simulink model "Model_with_decision"  (R2022a)
settings: Solver=VariableStepAuto  StartTime=0.0  StopTime=1000000  RelTol=1e-3
undefined symbols (not defined in the file): Coefficient_value, Enable_X, Enable_Y, N, s1, s10, s11, s12, s13, s14, s15, s16, s17, s18, s19, s2, s20, s21, s22, s23, s24, s25, s26, s27, s28, s29, s3, s30, s4, s5, s6, s7, s8, s9
libraries: simulink x35
(part 2 of 5)

== system Model_with_decision/Pbit_14 ==
  note: so EN=0 block simply passes the same OUT value to a multiport switch
  note: random value does not change when EN=0
  note: without a delay block, this block naturally gets the output of EN=1 block's output @ EN=0 so an unit delay is naturally applied
  IN : Inport
  EN : Inport  Port=2
  Cast To Double : DataTypeConversion  OutDataTypeStr=double  SaturateOnIntegerOverflow=off  RndMeth=Floor
  Cast To Double1 : DataTypeConversion  OutDataTypeStr=double  SaturateOnIntegerOverflow=off  RndMeth=Floor
  EN=0 Block : Subsystem  TreatAsAtomicUnit=on
  EN=1 Block : Subsystem  TreatAsAtomicUnit=on
  If : If
  Multiport Switch : MultiPortSwitch  DataPortOrder=Zero-based contiguous  Inputs=2  zeroidx=on  SaturateOnIntegerOverflow=off  InputSameDT=off
  OUT : Outport
  wires:
  IN/1 -> EN=1 Block/1(IN)
  EN/1 -> [EN], If/1
  Multiport Switch/1 -> OUT/1  "OUT_MUX"
  If/1 -> EN=1 Block/Action
  If/2 -> EN=0 Block/Action
  EN=1 Block/1(OUT) -> Cast To Double/1, EN=0 Block/1(IN)  "OUT_EN=1"
  EN=0 Block/1(Out1) -> Cast To Double1/1  "OUT_EN=0"
  [EN] -> Multiport Switch/1
  Cast To Double/1 -> Multiport Switch/3
  Cast To Double1/1 -> Multiport Switch/2

== system Model_with_decision/Pbit_15 ==
  note: without a delay block, this block naturally gets the output of EN=1 block's output @ EN=0 so an unit delay is naturally applied
  note: random value does not change when EN=0
  note: so EN=0 block simply passes the same OUT value to a multiport switch
  IN : Inport
  EN : Inport  Port=2
  Cast To Double : DataTypeConversion  OutDataTypeStr=double  SaturateOnIntegerOverflow=off  RndMeth=Floor
  Cast To Double1 : DataTypeConversion  OutDataTypeStr=double  SaturateOnIntegerOverflow=off  RndMeth=Floor
  EN=0 Block : Subsystem  TreatAsAtomicUnit=on
  EN=1 Block : Subsystem  TreatAsAtomicUnit=on
  If : If
  Multiport Switch : MultiPortSwitch  DataPortOrder=Zero-based contiguous  Inputs=2  zeroidx=on  SaturateOnIntegerOverflow=off  InputSameDT=off
  OUT : Outport
  wires:
  Cast To Double1/1 -> Multiport Switch/2
  Cast To Double/1 -> Multiport Switch/3
  [EN] -> Multiport Switch/1
  EN=0 Block/1(Out1) -> Cast To Double1/1  "OUT_EN=0"
  EN=1 Block/1(OUT) -> EN=0 Block/1(IN), Cast To Double/1  "OUT_EN=1"
  If/2 -> EN=0 Block/Action
  If/1 -> EN=1 Block/Action
  Multiport Switch/1 -> OUT/1  "OUT_MUX"
  EN/1 -> If/1, [EN]
  IN/1 -> EN=1 Block/1(IN)

== system Model_with_decision/Pbit_2 ==
  note: without a delay block, this block naturally gets the output of EN=1 block's output @ EN=0 so an unit delay is naturally applied
  note: random value does not change when EN=0
  note: so EN=0 block simply passes the same OUT value to a multiport switch
  IN : Inport
  EN : Inport  Port=2
  Cast To Double : DataTypeConversion  OutDataTypeStr=double  SaturateOnIntegerOverflow=off  RndMeth=Floor
  Cast To Double1 : DataTypeConversion  OutDataTypeStr=double  SaturateOnIntegerOverflow=off  RndMeth=Floor
  EN=0 Block : Subsystem  TreatAsAtomicUnit=on
  EN=1 Block : Subsystem  TreatAsAtomicUnit=on
  If : If
  Multiport Switch : MultiPortSwitch  DataPortOrder=Zero-based contiguous  Inputs=2  zeroidx=on  SaturateOnIntegerOverflow=off  InputSameDT=off
  OUT : Outport
  wires:
  Cast To Double1/1 -> Multiport Switch/2
  Cast To Double/1 -> Multiport Switch/3
  [EN] -> Multiport Switch/1
  EN=0 Block/1(Out1) -> Cast To Double1/1  "OUT_EN=0"
  EN=1 Block/1(OUT) -> EN=0 Block/1(IN), Cast To Double/1  "OUT_EN=1"
  If/2 -> EN=0 Block/Action
  If/1 -> EN=1 Block/Action
  Multiport Switch/1 -> OUT/1  "OUT_MUX"
  EN/1 -> If/1, [EN]
  IN/1 -> EN=1 Block/1(IN)

== system Model_with_decision/Pbit_3 ==
  note: so EN=0 block simply passes the same OUT value to a multiport switch
  note: random value does not change when EN=0
  note: without a delay block, this block naturally gets the output of EN=1 block's output @ EN=0 so an unit delay is naturally applied
  IN : Inport
  EN : Inport  Port=2
  Cast To Double : DataTypeConversion  OutDataTypeStr=double  SaturateOnIntegerOverflow=off  RndMeth=Floor
  Cast To Double1 : DataTypeConversion  OutDataTypeStr=double  SaturateOnIntegerOverflow=off  RndMeth=Floor
  EN=0 Block : Subsystem  TreatAsAtomicUnit=on
  EN=1 Block : Subsystem  TreatAsAtomicUnit=on
  If : If
  Multiport Switch : MultiPortSwitch  DataPortOrder=Zero-based contiguous  Inputs=2  zeroidx=on  SaturateOnIntegerOverflow=off  InputSameDT=off
  OUT : Outport
  wires:
  IN/1 -> EN=1 Block/1(IN)
  EN/1 -> [EN], If/1
  Multiport Switch/1 -> OUT/1  "OUT_MUX"
  If/1 -> EN=1 Block/Action
  If/2 -> EN=0 Block/Action
  EN=1 Block/1(OUT) -> Cast To Double/1, EN=0 Block/1(IN)  "OUT_EN=1"
  EN=0 Block/1(Out1) -> Cast To Double1/1  "OUT_EN=0"
  [EN] -> Multiport Switch/1
  Cast To Double/1 -> Multiport Switch/3
  Cast To Double1/1 -> Multiport Switch/2

== system Model_with_decision/Pbit_4 ==
  note: so EN=0 block simply passes the same OUT value to a multiport switch
  note: random value does not change when EN=0
  note: without a delay block, this block naturally gets the output of EN=1 block's output @ EN=0 so an unit delay is naturally applied
  IN : Inport
  EN : Inport  Port=2
  Cast To Double : DataTypeConversion  OutDataTypeStr=double  SaturateOnIntegerOverflow=off  RndMeth=Floor
  Cast To Double1 : DataTypeConversion  OutDataTypeStr=double  SaturateOnIntegerOverflow=off  RndMeth=Floor
  EN=0 Block : Subsystem  TreatAsAtomicUnit=on
  EN=1 Block : Subsystem  TreatAsAtomicUnit=on
  If : If
  Multiport Switch : MultiPortSwitch  DataPortOrder=Zero-based contiguous  Inputs=2  zeroidx=on  SaturateOnIntegerOverflow=off  InputSameDT=off
  OUT : Outport
  wires:
  IN/1 -> EN=1 Block/1(IN)
  EN/1 -> [EN], If/1
  Multiport Switch/1 -> OUT/1  "OUT_MUX"
  If/1 -> EN=1 Block/Action
  If/2 -> EN=0 Block/Action
  EN=1 Block/1(OUT) -> Cast To Double/1, EN=0 Block/1(IN)  "OUT_EN=1"
  EN=0 Block/1(Out1) -> Cast To Double1/1  "OUT_EN=0"
  [EN] -> Multiport Switch/1
  Cast To Double/1 -> Multiport Switch/3
  Cast To Double1/1 -> Multiport Switch/2

== system Model_with_decision/Pbit_5 ==
  note: without a delay block, this block naturally gets the output of EN=1 block's output @ EN=0 so an unit delay is naturally applied
  note: random value does not change when EN=0
  note: so EN=0 block simply passes the same OUT value to a multiport switch
  IN : Inport
  EN : Inport  Port=2
  Cast To Double : DataTypeConversion  OutDataTypeStr=double  SaturateOnIntegerOverflow=off  RndMeth=Floor
  Cast To Double1 : DataTypeConversion  OutDataTypeStr=double  SaturateOnIntegerOverflow=off  RndMeth=Floor
  EN=0 Block : Subsystem  TreatAsAtomicUnit=on
  EN=1 Block : Subsystem  TreatAsAtomicUnit=on
  If : If
  Multiport Switch : MultiPortSwitch  DataPortOrder=Zero-based contiguous  Inputs=2  zeroidx=on  SaturateOnIntegerOverflow=off  InputSameDT=off
  OUT : Outport
  wires:
  Cast To Double1/1 -> Multiport Switch/2
  Cast To Double/1 -> Multiport Switch/3
  [EN] -> Multiport Switch/1
  EN=0 Block/1(Out1) -> Cast To Double1/1  "OUT_EN=0"
  EN=1 Block/1(OUT) -> EN=0 Block/1(IN), Cast To Double/1  "OUT_EN=1"
  If/2 -> EN=0 Block/Action
  If/1 -> EN=1 Block/Action
  Multiport Switch/1 -> OUT/1  "OUT_MUX"
  EN/1 -> If/1, [EN]
  IN/1 -> EN=1 Block/1(IN)

== system Model_with_decision/Pbit_6 ==
  note: without a delay block, this block naturally gets the output of EN=1 block's output @ EN=0 so an unit delay is naturally applied
  note: random value does not change when EN=0
  note: so EN=0 block simply passes the same OUT value to a multiport switch
  IN : Inport
  EN : Inport  Port=2
  Cast To Double : DataTypeConversion  OutDataTypeStr=double  SaturateOnIntegerOverflow=off  RndMeth=Floor
  Cast To Double1 : DataTypeConversion  OutDataTypeStr=double  SaturateOnIntegerOverflow=off  RndMeth=Floor
  EN=0 Block : Subsystem  TreatAsAtomicUnit=on
  EN=1 Block : Subsystem  TreatAsAtomicUnit=on
  If : If
  Multiport Switch : MultiPortSwitch  DataPortOrder=Zero-based contiguous  Inputs=2  zeroidx=on  SaturateOnIntegerOverflow=off  InputSameDT=off
  OUT : Outport
  wires:
  Cast To Double1/1 -> Multiport Switch/2
  Cast To Double/1 -> Multiport Switch/3
  [EN] -> Multiport Switch/1
  EN=0 Block/1(Out1) -> Cast To Double1/1  "OUT_EN=0"
  EN=1 Block/1(OUT) -> EN=0 Block/1(IN), Cast To Double/1  "OUT_EN=1"
  If/2 -> EN=0 Block/Action
  If/1 -> EN=1 Block/Action
  Multiport Switch/1 -> OUT/1  "OUT_MUX"
  EN/1 -> If/1, [EN]
  IN/1 -> EN=1 Block/1(IN)

== system Model_with_decision/Pbit_7 ==
  note: without a delay block, this block naturally gets the output of EN=1 block's output @ EN=0 so an unit delay is naturally applied
  note: random value does not change when EN=0
  note: so EN=0 block simply passes the same OUT value to a multiport switch
  IN : Inport
  EN : Inport  Port=2
  Cast To Double : DataTypeConversion  OutDataTypeStr=double  SaturateOnIntegerOverflow=off  RndMeth=Floor
  Cast To Double1 : DataTypeConversion  OutDataTypeStr=double  SaturateOnIntegerOverflow=off  RndMeth=Floor
  EN=0 Block : Subsystem  TreatAsAtomicUnit=on
  EN=1 Block : Subsystem  TreatAsAtomicUnit=on
  If : If
  Multiport Switch : MultiPortSwitch  DataPortOrder=Zero-based contiguous  Inputs=2  zeroidx=on  SaturateOnIntegerOverflow=off  InputSameDT=off
  OUT : Outport
  wires:
  Cast To Double1/1 -> Multiport Switch/2
  Cast To Double/1 -> Multiport Switch/3
  [EN] -> Multiport Switch/1
  EN=0 Block/1(Out1) -> Cast To Double1/1  "OUT_EN=0"
  EN=1 Block/1(OUT) -> EN=0 Block/1(IN), Cast To Double/1  "OUT_EN=1"
  If/2 -> EN=0 Block/Action
  If/1 -> EN=1 Block/Action
  Multiport Switch/1 -> OUT/1  "OUT_MUX"
  EN/1 -> If/1, [EN]
  IN/1 -> EN=1 Block/1(IN)

== system Model_with_decision/Pbit_8 ==
  note: so EN=0 block simply passes the same OUT value to a multiport switch
  note: random value does not change when EN=0
  note: without a delay block, this block naturally gets the output of EN=1 block's output @ EN=0 so an unit delay is naturally applied
  IN : Inport
  EN : Inport  Port=2
  Cast To Double : DataTypeConversion  OutDataTypeStr=double  SaturateOnIntegerOverflow=off  RndMeth=Floor
  Cast To Double1 : DataTypeConversion  OutDataTypeStr=double  SaturateOnIntegerOverflow=off  RndMeth=Floor
  EN=0 Block : Subsystem  TreatAsAtomicUnit=on
  EN=1 Block : Subsystem  TreatAsAtomicUnit=on
  If : If
  Multiport Switch : MultiPortSwitch  DataPortOrder=Zero-based contiguous  Inputs=2  zeroidx=on  SaturateOnIntegerOverflow=off  InputSameDT=off
  OUT : Outport
  wires:
  IN/1 -> EN=1 Block/1(IN)
  EN/1 -> [EN], If/1
  Multiport Switch/1 -> OUT/1  "OUT_MUX"
  If/1 -> EN=1 Block/Action
  If/2 -> EN=0 Block/Action
  EN=1 Block/1(OUT) -> Cast To Double/1, EN=0 Block/1(IN)  "OUT_EN=1"
  EN=0 Block/1(Out1) -> Cast To Double1/1  "OUT_EN=0"
  [EN] -> Multiport Switch/1
  Cast To Double/1 -> Multiport Switch/3
  Cast To Double1/1 -> Multiport Switch/2

== system Model_with_decision/Pbit_9 ==
  note: so EN=0 block simply passes the same OUT value to a multiport switch
  note: random value does not change when EN=0
  note: without a delay block, this block naturally gets the output of EN=1 block's output @ EN=0 so an unit delay is naturally applied
  IN : Inport
  EN : Inport  Port=2
  Cast To Double : DataTypeConversion  OutDataTypeStr=double  SaturateOnIntegerOverflow=off  RndMeth=Floor
  Cast To Double1 : DataTypeConversion  OutDataTypeStr=double  SaturateOnIntegerOverflow=off  RndMeth=Floor
  EN=0 Block : Subsystem  TreatAsAtomicUnit=on
  EN=1 Block : Subsystem  TreatAsAtomicUnit=on
  If : If
  Multiport Switch : MultiPortSwitch  DataPortOrder=Zero-based contiguous  Inputs=2  zeroidx=on  SaturateOnIntegerOverflow=off  InputSameDT=off
  OUT : Outport
  wires:
  IN/1 -> EN=1 Block/1(IN)
  EN/1 -> [EN], If/1
  Multiport Switch/1 -> OUT/1  "OUT_MUX"
  If/1 -> EN=1 Block/Action
  If/2 -> EN=0 Block/Action
  EN=1 Block/1(OUT) -> Cast To Double/1, EN=0 Block/1(IN)  "OUT_EN=1"
  EN=0 Block/1(Out1) -> Cast To Double1/1  "OUT_EN=0"
  [EN] -> Multiport Switch/1
  Cast To Double/1 -> Multiport Switch/3
  Cast To Double1/1 -> Multiport Switch/2

== system Model_with_decision/Pbit_Y_1 ==
  note: without a delay block, this block naturally gets the output of EN=1 block's output @ EN=0 so an unit delay is naturally applied
  note: random value does not change when EN=0
  note: so EN=0 block simply passes the same OUT value to a multiport switch
  IN : Inport
  EN : Inport  Port=2
  Cast To Double : DataTypeConversion  OutDataTypeStr=double  SaturateOnIntegerOverflow=off  RndMeth=Floor
  Cast To Double1 : DataTypeConversion  OutDataTypeStr=double  SaturateOnIntegerOverflow=off  RndMeth=Floor
  EN=0 Block : Subsystem  TreatAsAtomicUnit=on
  EN=1 Block : Subsystem  TreatAsAtomicUnit=on
  If : If
  Multiport Switch : MultiPortSwitch  DataPortOrder=Zero-based contiguous  Inputs=2  zeroidx=on  SaturateOnIntegerOverflow=off  InputSameDT=off
  OUT : Outport
  wires:
  Cast To Double1/1 -> Multiport Switch/2
  Cast To Double/1 -> Multiport Switch/3
  [EN] -> Multiport Switch/1
  EN=0 Block/1(Out1) -> Cast To Double1/1  "OUT_EN=0"
  EN=1 Block/1(OUT) -> EN=0 Block/1(IN), Cast To Double/1  "OUT_EN=1"
  If/2 -> EN=0 Block/Action
  If/1 -> EN=1 Block/Action
  Multiport Switch/1 -> OUT/1  "OUT_MUX"
  EN/1 -> If/1, [EN]
  IN/1 -> EN=1 Block/1(IN)

== system Model_with_decision/Pbit_Y_10 ==
  note: without a delay block, this block naturally gets the output of EN=1 block's output @ EN=0 so an unit delay is naturally applied
  note: random value does not change when EN=0
  note: so EN=0 block simply passes the same OUT value to a multiport switch
  IN : Inport
  EN : Inport  Port=2
  Cast To Double : DataTypeConversion  OutDataTypeStr=double  SaturateOnIntegerOverflow=off  RndMeth=Floor
  Cast To Double1 : DataTypeConversion  OutDataTypeStr=double  SaturateOnIntegerOverflow=off  RndMeth=Floor
  EN=0 Block : Subsystem  TreatAsAtomicUnit=on
  EN=1 Block : Subsystem  TreatAsAtomicUnit=on
  If : If
  Multiport Switch : MultiPortSwitch  DataPortOrder=Zero-based contiguous  Inputs=2  zeroidx=on  SaturateOnIntegerOverflow=off  InputSameDT=off
  OUT : Outport
  wires:
  Cast To Double1/1 -> Multiport Switch/2
  Cast To Double/1 -> Multiport Switch/3
  [EN] -> Multiport Switch/1
  EN=0 Block/1(Out1) -> Cast To Double1/1  "OUT_EN=0"
  EN=1 Block/1(OUT) -> EN=0 Block/1(IN), Cast To Double/1  "OUT_EN=1"
  If/2 -> EN=0 Block/Action
  If/1 -> EN=1 Block/Action
  Multiport Switch/1 -> OUT/1  "OUT_MUX"
  EN/1 -> If/1, [EN]
  IN/1 -> EN=1 Block/1(IN)

== system Model_with_decision/Pbit_Y_11 ==
  note: without a delay block, this block naturally gets the output of EN=1 block's output @ EN=0 so an unit delay is naturally applied
  note: random value does not change when EN=0
  note: so EN=0 block simply passes the same OUT value to a multiport switch
  IN : Inport
  EN : Inport  Port=2
  Cast To Double : DataTypeConversion  OutDataTypeStr=double  SaturateOnIntegerOverflow=off  RndMeth=Floor
  Cast To Double1 : DataTypeConversion  OutDataTypeStr=double  SaturateOnIntegerOverflow=off  RndMeth=Floor
  EN=0 Block : Subsystem  TreatAsAtomicUnit=on
  EN=1 Block : Subsystem  TreatAsAtomicUnit=on
  If : If
  Multiport Switch : MultiPortSwitch  DataPortOrder=Zero-based contiguous  Inputs=2  zeroidx=on  SaturateOnIntegerOverflow=off  InputSameDT=off
  OUT : Outport
  wires:
  Cast To Double1/1 -> Multiport Switch/2
  Cast To Double/1 -> Multiport Switch/3
  [EN] -> Multiport Switch/1
  EN=0 Block/1(Out1) -> Cast To Double1/1  "OUT_EN=0"
  EN=1 Block/1(OUT) -> EN=0 Block/1(IN), Cast To Double/1  "OUT_EN=1"
  If/2 -> EN=0 Block/Action
  If/1 -> EN=1 Block/Action
  Multiport Switch/1 -> OUT/1  "OUT_MUX"
  EN/1 -> If/1, [EN]
  IN/1 -> EN=1 Block/1(IN)

== system Model_with_decision/Pbit_Y_12 ==
  note: without a delay block, this block naturally gets the output of EN=1 block's output @ EN=0 so an unit delay is naturally applied
  note: random value does not change when EN=0
  note: so EN=0 block simply passes the same OUT value to a multiport switch
  IN : Inport
  EN : Inport  Port=2
  Cast To Double : DataTypeConversion  OutDataTypeStr=double  SaturateOnIntegerOverflow=off  RndMeth=Floor
  Cast To Double1 : DataTypeConversion  OutDataTypeStr=double  SaturateOnIntegerOverflow=off  RndMeth=Floor
  EN=0 Block : Subsystem  TreatAsAtomicUnit=on
  EN=1 Block : Subsystem  TreatAsAtomicUnit=on
  If : If
  Multiport Switch : MultiPortSwitch  DataPortOrder=Zero-based contiguous  Inputs=2  zeroidx=on  SaturateOnIntegerOverflow=off  InputSameDT=off
  OUT : Outport
  wires:
  Cast To Double1/1 -> Multiport Switch/2
  Cast To Double/1 -> Multiport Switch/3
  [EN] -> Multiport Switch/1
  EN=0 Block/1(Out1) -> Cast To Double1/1  "OUT_EN=0"
  EN=1 Block/1(OUT) -> EN=0 Block/1(IN), Cast To Double/1  "OUT_EN=1"
  If/2 -> EN=0 Block/Action
  If/1 -> EN=1 Block/Action
  Multiport Switch/1 -> OUT/1  "OUT_MUX"
  EN/1 -> If/1, [EN]
  IN/1 -> EN=1 Block/1(IN)

== system Model_with_decision/Pbit_Y_13 ==
  note: so EN=0 block simply passes the same OUT value to a multiport switch
  note: random value does not change when EN=0
  note: without a delay block, this block naturally gets the output of EN=1 block's output @ EN=0 so an unit delay is naturally applied
  IN : Inport
  EN : Inport  Port=2
  Cast To Double : DataTypeConversion  OutDataTypeStr=double  SaturateOnIntegerOverflow=off  RndMeth=Floor
  Cast To Double1 : DataTypeConversion  OutDataTypeStr=double  SaturateOnIntegerOverflow=off  RndMeth=Floor
  EN=0 Block : Subsystem  TreatAsAtomicUnit=on
  EN=1 Block : Subsystem  TreatAsAtomicUnit=on
  If : If
  Multiport Switch : MultiPortSwitch  DataPortOrder=Zero-based contiguous  Inputs=2  zeroidx=on  SaturateOnIntegerOverflow=off  InputSameDT=off
  OUT : Outport
  wires:
  IN/1 -> EN=1 Block/1(IN)
  EN/1 -> [EN], If/1
  Multiport Switch/1 -> OUT/1  "OUT_MUX"
  If/1 -> EN=1 Block/Action
  If/2 -> EN=0 Block/Action
  EN=1 Block/1(OUT) -> Cast To Double/1, EN=0 Block/1(IN)  "OUT_EN=1"
  EN=0 Block/1(Out1) -> Cast To Double1/1  "OUT_EN=0"
  [EN] -> Multiport Switch/1
  Cast To Double/1 -> Multiport Switch/3
  Cast To Double1/1 -> Multiport Switch/2

== system Model_with_decision/Pbit_Y_14 ==
  note: so EN=0 block simply passes the same OUT value to a multiport switch
  note: random value does not change when EN=0
  note: without a delay block, this block naturally gets the output of EN=1 block's output @ EN=0 so an unit delay is naturally applied
  IN : Inport
  EN : Inport  Port=2
  Cast To Double : DataTypeConversion  OutDataTypeStr=double  SaturateOnIntegerOverflow=off  RndMeth=Floor
  Cast To Double1 : DataTypeConversion  OutDataTypeStr=double  SaturateOnIntegerOverflow=off  RndMeth=Floor
  EN=0 Block : Subsystem  TreatAsAtomicUnit=on
  EN=1 Block : Subsystem  TreatAsAtomicUnit=on
  If : If
  Multiport Switch : MultiPortSwitch  DataPortOrder=Zero-based contiguous  Inputs=2  zeroidx=on  SaturateOnIntegerOverflow=off  InputSameDT=off
  OUT : Outport
  wires:
  IN/1 -> EN=1 Block/1(IN)
  EN/1 -> [EN], If/1
  Multiport Switch/1 -> OUT/1  "OUT_MUX"
  If/1 -> EN=1 Block/Action
  If/2 -> EN=0 Block/Action
  EN=1 Block/1(OUT) -> Cast To Double/1, EN=0 Block/1(IN)  "OUT_EN=1"
  EN=0 Block/1(Out1) -> Cast To Double1/1  "OUT_EN=0"
  [EN] -> Multiport Switch/1
  Cast To Double/1 -> Multiport Switch/3
  Cast To Double1/1 -> Multiport Switch/2

== system Model_with_decision/Pbit_Y_15 ==
  note: so EN=0 block simply passes the same OUT value to a multiport switch
  note: random value does not change when EN=0
  note: without a delay block, this block naturally gets the output of EN=1 block's output @ EN=0 so an unit delay is naturally applied
  IN : Inport
  EN : Inport  Port=2
  Cast To Double : DataTypeConversion  OutDataTypeStr=double  SaturateOnIntegerOverflow=off  RndMeth=Floor
  Cast To Double1 : DataTypeConversion  OutDataTypeStr=double  SaturateOnIntegerOverflow=off  RndMeth=Floor
  EN=0 Block : Subsystem  TreatAsAtomicUnit=on
  EN=1 Block : Subsystem  TreatAsAtomicUnit=on
  If : If
  Multiport Switch : MultiPortSwitch  DataPortOrder=Zero-based contiguous  Inputs=2  zeroidx=on  SaturateOnIntegerOverflow=off  InputSameDT=off
  OUT : Outport
  wires:
  IN/1 -> EN=1 Block/1(IN)
  EN/1 -> [EN], If/1
  Multiport Switch/1 -> OUT/1  "OUT_MUX"
  If/1 -> EN=1 Block/Action
  If/2 -> EN=0 Block/Action
  EN=1 Block/1(OUT) -> Cast To Double/1, EN=0 Block/1(IN)  "OUT_EN=1"
  EN=0 Block/1(Out1) -> Cast To Double1/1  "OUT_EN=0"
  [EN] -> Multiport Switch/1
  Cast To Double/1 -> Multiport Switch/3
  Cast To Double1/1 -> Multiport Switch/2

== system Model_with_decision/Pbit_Y_2 ==
  note: without a delay block, this block naturally gets the output of EN=1 block's output @ EN=0 so an unit delay is naturally applied
  note: random value does not change when EN=0
  note: so EN=0 block simply passes the same OUT value to a multiport switch
  IN : Inport
  EN : Inport  Port=2
  Cast To Double : DataTypeConversion  OutDataTypeStr=double  SaturateOnIntegerOverflow=off  RndMeth=Floor
  Cast To Double1 : DataTypeConversion  OutDataTypeStr=double  SaturateOnIntegerOverflow=off  RndMeth=Floor
  EN=0 Block : Subsystem  TreatAsAtomicUnit=on
  EN=1 Block : Subsystem  TreatAsAtomicUnit=on
  If : If
  Multiport Switch : MultiPortSwitch  DataPortOrder=Zero-based contiguous  Inputs=2  zeroidx=on  SaturateOnIntegerOverflow=off  InputSameDT=off
  OUT : Outport
  wires:
  Cast To Double1/1 -> Multiport Switch/2
  Cast To Double/1 -> Multiport Switch/3
  [EN] -> Multiport Switch/1
  EN=0 Block/1(Out1) -> Cast To Double1/1  "OUT_EN=0"
  EN=1 Block/1(OUT) -> EN=0 Block/1(IN), Cast To Double/1  "OUT_EN=1"
  If/2 -> EN=0 Block/Action
  If/1 -> EN=1 Block/Action
  Multiport Switch/1 -> OUT/1  "OUT_MUX"
  EN/1 -> If/1, [EN]
  IN/1 -> EN=1 Block/1(IN)

== system Model_with_decision/Pbit_Y_3 ==
  note: so EN=0 block simply passes the same OUT value to a multiport switch
  note: random value does not change when EN=0
  note: without a delay block, this block naturally gets the output of EN=1 block's output @ EN=0 so an unit delay is naturally applied
  IN : Inport
  EN : Inport  Port=2
  Cast To Double : DataTypeConversion  OutDataTypeStr=double  SaturateOnIntegerOverflow=off  RndMeth=Floor
  Cast To Double1 : DataTypeConversion  OutDataTypeStr=double  SaturateOnIntegerOverflow=off  RndMeth=Floor
  EN=0 Block : Subsystem  TreatAsAtomicUnit=on
  EN=1 Block : Subsystem  TreatAsAtomicUnit=on
  If : If
  Multiport Switch : MultiPortSwitch  DataPortOrder=Zero-based contiguous  Inputs=2  zeroidx=on  SaturateOnIntegerOverflow=off  InputSameDT=off
  OUT : Outport
  wires:
  IN/1 -> EN=1 Block/1(IN)
  EN/1 -> [EN], If/1
  Multiport Switch/1 -> OUT/1  "OUT_MUX"
  If/1 -> EN=1 Block/Action
  If/2 -> EN=0 Block/Action
  EN=1 Block/1(OUT) -> Cast To Double/1, EN=0 Block/1(IN)  "OUT_EN=1"
  EN=0 Block/1(Out1) -> Cast To Double1/1  "OUT_EN=0"
  [EN] -> Multiport Switch/1
  Cast To Double/1 -> Multiport Switch/3
  Cast To Double1/1 -> Multiport Switch/2

== system Model_with_decision/Pbit_Y_4 ==
  note: so EN=0 block simply passes the same OUT value to a multiport switch
  note: random value does not change when EN=0
  note: without a delay block, this block naturally gets the output of EN=1 block's output @ EN=0 so an unit delay is naturally applied
  IN : Inport
  EN : Inport  Port=2
  Cast To Double : DataTypeConversion  OutDataTypeStr=double  SaturateOnIntegerOverflow=off  RndMeth=Floor
  Cast To Double1 : DataTypeConversion  OutDataTypeStr=double  SaturateOnIntegerOverflow=off  RndMeth=Floor
  EN=0 Block : Subsystem  TreatAsAtomicUnit=on
  EN=1 Block : Subsystem  TreatAsAtomicUnit=on
  If : If
  Multiport Switch : MultiPortSwitch  DataPortOrder=Zero-based contiguous  Inputs=2  zeroidx=on  SaturateOnIntegerOverflow=off  InputSameDT=off
  OUT : Outport
  wires:
  IN/1 -> EN=1 Block/1(IN)
  EN/1 -> [EN], If/1
  Multiport Switch/1 -> OUT/1  "OUT_MUX"
  If/1 -> EN=1 Block/Action
  If/2 -> EN=0 Block/Action
  EN=1 Block/1(OUT) -> Cast To Double/1, EN=0 Block/1(IN)  "OUT_EN=1"
  EN=0 Block/1(Out1) -> Cast To Double1/1  "OUT_EN=0"
  [EN] -> Multiport Switch/1
  Cast To Double/1 -> Multiport Switch/3
  Cast To Double1/1 -> Multiport Switch/2

== system Model_with_decision/Pbit_Y_5 ==
  note: without a delay block, this block naturally gets the output of EN=1 block's output @ EN=0 so an unit delay is naturally applied
  note: random value does not change when EN=0
  note: so EN=0 block simply passes the same OUT value to a multiport switch
  IN : Inport
  EN : Inport  Port=2
  Cast To Double : DataTypeConversion  OutDataTypeStr=double  SaturateOnIntegerOverflow=off  RndMeth=Floor
  Cast To Double1 : DataTypeConversion  OutDataTypeStr=double  SaturateOnIntegerOverflow=off  RndMeth=Floor
  EN=0 Block : Subsystem  TreatAsAtomicUnit=on
  EN=1 Block : Subsystem  TreatAsAtomicUnit=on
  If : If
  Multiport Switch : MultiPortSwitch  DataPortOrder=Zero-based contiguous  Inputs=2  zeroidx=on  SaturateOnIntegerOverflow=off  InputSameDT=off
  OUT : Outport
  wires:
  Cast To Double1/1 -> Multiport Switch/2
  Cast To Double/1 -> Multiport Switch/3
  [EN] -> Multiport Switch/1
  EN=0 Block/1(Out1) -> Cast To Double1/1  "OUT_EN=0"
  EN=1 Block/1(OUT) -> EN=0 Block/1(IN), Cast To Double/1  "OUT_EN=1"
  If/2 -> EN=0 Block/Action
  If/1 -> EN=1 Block/Action
  Multiport Switch/1 -> OUT/1  "OUT_MUX"
  EN/1 -> If/1, [EN]
  IN/1 -> EN=1 Block/1(IN)

== system Model_with_decision/Pbit_Y_6 ==
  note: without a delay block, this block naturally gets the output of EN=1 block's output @ EN=0 so an unit delay is naturally applied
  note: random value does not change when EN=0
  note: so EN=0 block simply passes the same OUT value to a multiport switch
  IN : Inport
  EN : Inport  Port=2
  Cast To Double : DataTypeConversion  OutDataTypeStr=double  SaturateOnIntegerOverflow=off  RndMeth=Floor
  Cast To Double1 : DataTypeConversion  OutDataTypeStr=double  SaturateOnIntegerOverflow=off  RndMeth=Floor
  EN=0 Block : Subsystem  TreatAsAtomicUnit=on
  EN=1 Block : Subsystem  TreatAsAtomicUnit=on
  If : If
  Multiport Switch : MultiPortSwitch  DataPortOrder=Zero-based contiguous  Inputs=2  zeroidx=on  SaturateOnIntegerOverflow=off  InputSameDT=off
  OUT : Outport
  wires:
  Cast To Double1/1 -> Multiport Switch/2
  Cast To Double/1 -> Multiport Switch/3
  [EN] -> Multiport Switch/1
  EN=0 Block/1(Out1) -> Cast To Double1/1  "OUT_EN=0"
  EN=1 Block/1(OUT) -> EN=0 Block/1(IN), Cast To Double/1  "OUT_EN=1"
  If/2 -> EN=0 Block/Action
  If/1 -> EN=1 Block/Action
  Multiport Switch/1 -> OUT/1  "OUT_MUX"
  EN/1 -> If/1, [EN]
  IN/1 -> EN=1 Block/1(IN)

== system Model_with_decision/Pbit_Y_7 ==
  note: without a delay block, this block naturally gets the output of EN=1 block's output @ EN=0 so an unit delay is naturally applied
  note: random value does not change when EN=0
  note: so EN=0 block simply passes the same OUT value to a multiport switch
  IN : Inport
  EN : Inport  Port=2
  Cast To Double : DataTypeConversion  OutDataTypeStr=double  SaturateOnIntegerOverflow=off  RndMeth=Floor
  Cast To Double1 : DataTypeConversion  OutDataTypeStr=double  SaturateOnIntegerOverflow=off  RndMeth=Floor
  EN=0 Block : Subsystem  TreatAsAtomicUnit=on
  EN=1 Block : Subsystem  TreatAsAtomicUnit=on
  If : If
  Multiport Switch : MultiPortSwitch  DataPortOrder=Zero-based contiguous  Inputs=2  zeroidx=on  SaturateOnIntegerOverflow=off  InputSameDT=off
  OUT : Outport
  wires:
  Cast To Double1/1 -> Multiport Switch/2
  Cast To Double/1 -> Multiport Switch/3
  [EN] -> Multiport Switch/1
  EN=0 Block/1(Out1) -> Cast To Double1/1  "OUT_EN=0"
  EN=1 Block/1(OUT) -> EN=0 Block/1(IN), Cast To Double/1  "OUT_EN=1"
  If/2 -> EN=0 Block/Action
  If/1 -> EN=1 Block/Action
  Multiport Switch/1 -> OUT/1  "OUT_MUX"
  EN/1 -> If/1, [EN]
  IN/1 -> EN=1 Block/1(IN)

== system Model_with_decision/Pbit_Y_8 ==
  note: so EN=0 block simply passes the same OUT value to a multiport switch
  note: random value does not change when EN=0
  note: without a delay block, this block naturally gets the output of EN=1 block's output @ EN=0 so an unit delay is naturally applied
  IN : Inport
  EN : Inport  Port=2
  Cast To Double : DataTypeConversion  OutDataTypeStr=double  SaturateOnIntegerOverflow=off  RndMeth=Floor
  Cast To Double1 : DataTypeConversion  OutDataTypeStr=double  SaturateOnIntegerOverflow=off  RndMeth=Floor
  EN=0 Block : Subsystem  TreatAsAtomicUnit=on
  EN=1 Block : Subsystem  TreatAsAtomicUnit=on
  If : If
  Multiport Switch : MultiPortSwitch  DataPortOrder=Zero-based contiguous  Inputs=2  zeroidx=on  SaturateOnIntegerOverflow=off  InputSameDT=off
  OUT : Outport
  wires:
  IN/1 -> EN=1 Block/1(IN)
  EN/1 -> [EN], If/1
  Multiport Switch/1 -> OUT/1  "OUT_MUX"
  If/1 -> EN=1 Block/Action
  If/2 -> EN=0 Block/Action
  EN=1 Block/1(OUT) -> Cast To Double/1, EN=0 Block/1(IN)  "OUT_EN=1"
  EN=0 Block/1(Out1) -> Cast To Double1/1  "OUT_EN=0"
  [EN] -> Multiport Switch/1
  Cast To Double/1 -> Multiport Switch/3
  Cast To Double1/1 -> Multiport Switch/2

== system Model_with_decision/Pbit_Y_9 ==
  note: so EN=0 block simply passes the same OUT value to a multiport switch
  note: random value does not change when EN=0
  note: without a delay block, this block naturally gets the output of EN=1 block's output @ EN=0 so an unit delay is naturally applied
  IN : Inport
  EN : Inport  Port=2
  Cast To Double : DataTypeConversion  OutDataTypeStr=double  SaturateOnIntegerOverflow=off  RndMeth=Floor
  Cast To Double1 : DataTypeConversion  OutDataTypeStr=double  SaturateOnIntegerOverflow=off  RndMeth=Floor
  EN=0 Block : Subsystem  TreatAsAtomicUnit=on
  EN=1 Block : Subsystem  TreatAsAtomicUnit=on
  If : If
  Multiport Switch : MultiPortSwitch  DataPortOrder=Zero-based contiguous  Inputs=2  zeroidx=on  SaturateOnIntegerOverflow=off  InputSameDT=off
  OUT : Outport
  wires:
  IN/1 -> EN=1 Block/1(IN)
  EN/1 -> [EN], If/1
  Multiport Switch/1 -> OUT/1  "OUT_MUX"
  If/1 -> EN=1 Block/Action
  If/2 -> EN=0 Block/Action
  EN=1 Block/1(OUT) -> Cast To Double/1, EN=0 Block/1(IN)  "OUT_EN=1"
  EN=0 Block/1(Out1) -> Cast To Double1/1  "OUT_EN=0"
  [EN] -> Multiport Switch/1
  Cast To Double/1 -> Multiport Switch/3
  Cast To Double1/1 -> Multiport Switch/2

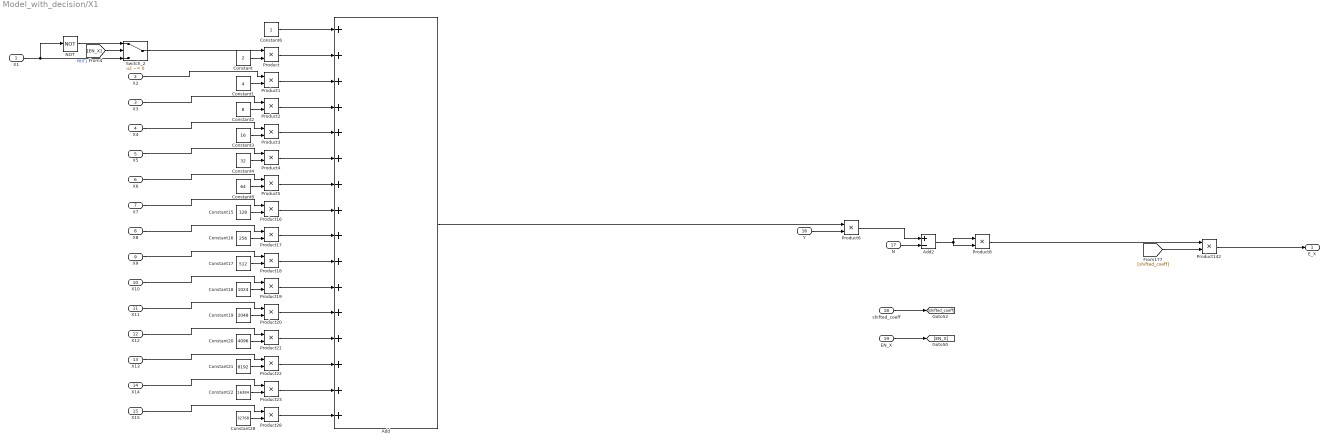
== system Model_with_decision/X1 ==
  X1 : Inport  OutDataTypeStr=fixdt(0,1,0)  LockScale=on
  X2 : Inport  Port=2  OutDataTypeStr=fixdt(0,1,0)  LockScale=on
  X3 : Inport  Port=3  OutDataTypeStr=fixdt(0,1,0)  LockScale=on
  X4 : Inport  Port=4  OutDataTypeStr=fixdt(0,1,0)  LockScale=on
  X5 : Inport  Port=5  OutDataTypeStr=fixdt(0,1,0)  LockScale=on
  X6 : Inport  Port=6  OutDataTypeStr=fixdt(0,1,0)  LockScale=on
  X7 : Inport  Port=7  OutDataTypeStr=fixdt(0,1,0)  LockScale=on
  X8 : Inport  Port=8  OutDataTypeStr=fixdt(0,1,0)  LockScale=on
  X9 : Inport  Port=9  OutDataTypeStr=fixdt(0,1,0)  LockScale=on
  X10 : Inport  Port=10  OutDataTypeStr=fixdt(0,1,0)  LockScale=on
  X11 : Inport  Port=11  OutDataTypeStr=fixdt(0,1,0)  LockScale=on
  X12 : Inport  Port=12  OutDataTypeStr=fixdt(0,1,0)  LockScale=on
  X13 : Inport  Port=13  OutDataTypeStr=fixdt(0,1,0)  LockScale=on
  X14 : Inport  Port=14  OutDataTypeStr=fixdt(0,1,0)  LockScale=on
  X15 : Inport  Port=15  OutDataTypeStr=fixdt(0,1,0)  LockScale=on
  Y : Inport  Port=16  LockScale=on
  N : Inport  Port=17  LockScale=on
  shifted_coeff : Inport  Port=18  LockScale=on
  EN_X : Inport  Port=19  OutDataTypeStr=fixdt(0,1,0)  LockScale=on
  Add : Sum  Inputs=++++++++++++++++
  Add2 : Sum  Inputs=+-
  Constant : Constant  Value=2
  Constant1 : Constant  Value=4
  Constant15 : Constant  Value=128
  Constant16 : Constant  Value=256
  Constant17 : Constant  Value=512
  Constant18 : Constant  Value=1024
  Constant19 : Constant  Value=2048
  Constant2 : Constant  Value=8
  Constant20 : Constant  Value=4096
  Constant21 : Constant  Value=8192
  Constant22 : Constant  Value=16384
  Constant28 : Constant  Value=32768
  Constant3 : Constant  Value=16
  Constant4 : Constant  Value=32
  Constant6 : Constant
  Constant8 : Constant  Value=64
  NOT : Logic  Operator=NOT  IconShape=distinctive  AllPortsSameDT=off  OutDataTypeStr=boolean
  Product{,1..6,8,16..23,28,142} (18 alike) : Product
  Switch_2 : Switch  Criteria=u2 ~= 0  OutDataTypeStr=fixdt(0,1,0)  SaturateOnIntegerOverflow=off  InputSameDT=off
  E_X : Outport  LockScale=on
  wires:
  Constant/1 -> Product/2
  Switch_2/1 -> Product/1
  Constant1/1 -> Product1/2
  X2/1 -> Product1/1
  Constant2/1 -> Product2/2
  X3/1 -> Product2/1
  Constant6/1 -> Add/1
  Product/1 -> Add/2
  Product1/1 -> Add/3
  Product2/1 -> Add/4
  Add/1 -> Product6/1
  Add2/1 -> Product8/2, Product8/1
  Product4/1 -> Add/6
  Constant4/1 -> Product4/2
  Constant8/1 -> Product5/2
  X6/1 -> Product5/1
  Product3/1 -> Add/5
  X4/1 -> Product3/1
  Product5/1 -> Add/7
  X5/1 -> Product4/1
  Constant3/1 -> Product3/2
  Product19/1 -> Add/11
  Constant20/1 -> Product21/2
  Constant18/1 -> Product19/2
  Product18/1 -> Add/10
  Constant15/1 -> Product16/2
  Constant16/1 -> Product17/2
  X11/1 -> Product20/1
  Product20/1 -> Add/12
  X8/1 -> Product17/1
  X10/1 -> Product19/1
  X7/1 -> Product16/1
  Constant19/1 -> Product20/2
  Product16/1 -> Add/8
  X9/1 -> Product18/1
  Constant17/1 -> Product18/2
  Product21/1 -> Add/13
  X12/1 -> Product21/1
  Product17/1 -> Add/9
  X14/1 -> Product23/1
  X15/1 -> Product28/1
  Constant28/1 -> Product28/2
  Product28/1 -> Add/16
  Product22/1 -> Add/14
  Product23/1 -> Add/15
  Constant21/1 -> Product22/2
  Constant22/1 -> Product23/2
  [EN_X] -> Switch_2/2
  X1/1 -> NOT/1, Switch_2/3  "PBIT1"
  NOT/1 -> Switch_2/1
  X13/1 -> Product22/1
  EN_X/1 -> [EN_X]
  shifted_coeff/1 -> [shifted_coeff]
  Product142/1 -> E_X/1
  [shifted_coeff] -> Product142/2
  Product6/1 -> Add2/1
  Product8/1 -> Product142/1
  N/1 -> Add2/2
  Y/1 -> Product6/2

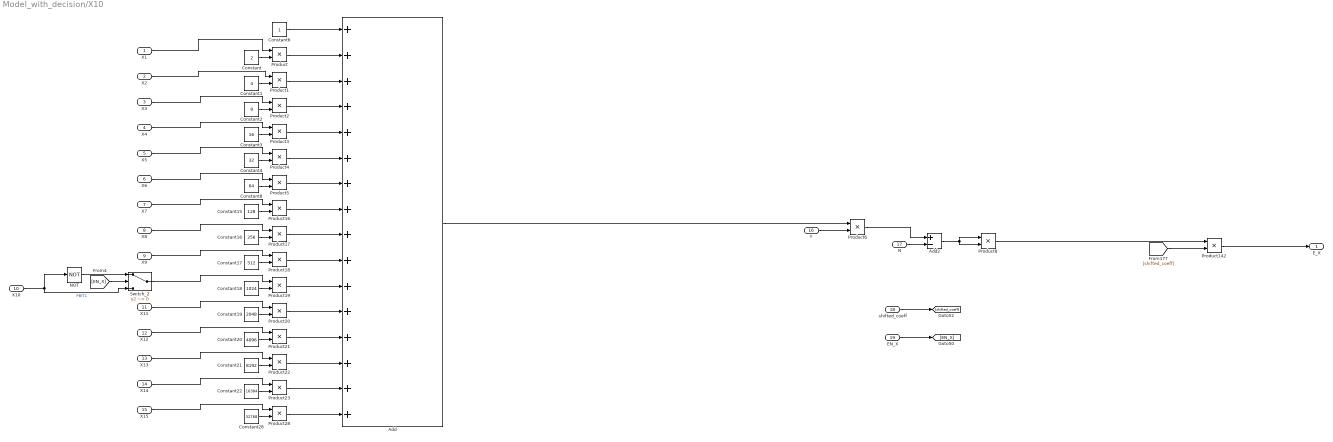
== system Model_with_decision/X10 ==
  X1 : Inport  OutDataTypeStr=fixdt(0,1,0)  LockScale=on
  X2 : Inport  Port=2  OutDataTypeStr=fixdt(0,1,0)  LockScale=on
  X3 : Inport  Port=3  OutDataTypeStr=fixdt(0,1,0)  LockScale=on
  X4 : Inport  Port=4  OutDataTypeStr=fixdt(0,1,0)  LockScale=on
  X5 : Inport  Port=5  OutDataTypeStr=fixdt(0,1,0)  LockScale=on
  X6 : Inport  Port=6  OutDataTypeStr=fixdt(0,1,0)  LockScale=on
  X7 : Inport  Port=7  OutDataTypeStr=fixdt(0,1,0)  LockScale=on
  X8 : Inport  Port=8  OutDataTypeStr=fixdt(0,1,0)  LockScale=on
  X9 : Inport  Port=9  OutDataTypeStr=fixdt(0,1,0)  LockScale=on
  X10 : Inport  Port=10  OutDataTypeStr=fixdt(0,1,0)  LockScale=on
  X11 : Inport  Port=11  OutDataTypeStr=fixdt(0,1,0)  LockScale=on
  X12 : Inport  Port=12  OutDataTypeStr=fixdt(0,1,0)  LockScale=on
  X13 : Inport  Port=13  OutDataTypeStr=fixdt(0,1,0)  LockScale=on
  X14 : Inport  Port=14  OutDataTypeStr=fixdt(0,1,0)  LockScale=on
  X15 : Inport  Port=15  OutDataTypeStr=fixdt(0,1,0)  LockScale=on
  Y : Inport  Port=16  LockScale=on
  N : Inport  Port=17  LockScale=on
  shifted_coeff : Inport  Port=18  LockScale=on
  EN_X : Inport  Port=19  OutDataTypeStr=fixdt(0,1,0)  LockScale=on
  Add : Sum  Inputs=++++++++++++++++
  Add2 : Sum  Inputs=+-
  Constant : Constant  Value=2
  Constant1 : Constant  Value=4
  Constant15 : Constant  Value=128
  Constant16 : Constant  Value=256
  Constant17 : Constant  Value=512
  Constant18 : Constant  Value=1024
  Constant19 : Constant  Value=2048
  Constant2 : Constant  Value=8
  Constant20 : Constant  Value=4096
  Constant21 : Constant  Value=8192
  Constant22 : Constant  Value=16384
  Constant28 : Constant  Value=32768
  Constant3 : Constant  Value=16
  Constant4 : Constant  Value=32
  Constant6 : Constant
  Constant8 : Constant  Value=64
  NOT : Logic  Operator=NOT  IconShape=distinctive  AllPortsSameDT=off  OutDataTypeStr=boolean
  Product{,1..6,8,16..23,28,142} (18 alike) : Product
  Switch_2 : Switch  Criteria=u2 ~= 0  OutDataTypeStr=fixdt(0,1,0)  SaturateOnIntegerOverflow=off  InputSameDT=off
  E_X : Outport  LockScale=on
  wires:
  Constant/1 -> Product/2
  X1/1 -> Product/1
  Constant1/1 -> Product1/2
  X2/1 -> Product1/1
  Constant2/1 -> Product2/2
  X3/1 -> Product2/1
  Constant6/1 -> Add/1
  Product/1 -> Add/2
  Product1/1 -> Add/3
  Product2/1 -> Add/4
  Add/1 -> Product6/1
  Add2/1 -> Product8/2, Product8/1
  Product4/1 -> Add/6
  Constant4/1 -> Product4/2
  Constant8/1 -> Product5/2
  X6/1 -> Product5/1
  Product3/1 -> Add/5
  X4/1 -> Product3/1
  Product5/1 -> Add/7
  X5/1 -> Product4/1
  Constant3/1 -> Product3/2
  Product19/1 -> Add/11
  Constant20/1 -> Product21/2
  Constant18/1 -> Product19/2
  Product18/1 -> Add/10
  Constant15/1 -> Product16/2
  Constant16/1 -> Product17/2
  X11/1 -> Product20/1
  Product20/1 -> Add/12
  X8/1 -> Product17/1
  Switch_2/1 -> Product19/1
  X7/1 -> Product16/1
  Constant19/1 -> Product20/2
  Product16/1 -> Add/8
  X9/1 -> Product18/1
  Constant17/1 -> Product18/2
  Product21/1 -> Add/13
  X12/1 -> Product21/1
  Product17/1 -> Add/9
  X14/1 -> Product23/1
  X15/1 -> Product28/1
  Constant28/1 -> Product28/2
  Product28/1 -> Add/16
  Product22/1 -> Add/14
  Product23/1 -> Add/15
  Constant21/1 -> Product22/2
  Constant22/1 -> Product23/2
  [EN_X] -> Switch_2/2
  X10/1 -> NOT/1, Switch_2/3  "PBIT1"
  NOT/1 -> Switch_2/1
  X13/1 -> Product22/1
  EN_X/1 -> [EN_X]
  shifted_coeff/1 -> [shifted_coeff]
  Product142/1 -> E_X/1
  [shifted_coeff] -> Product142/2
  Product6/1 -> Add2/1
  Product8/1 -> Product142/1
  N/1 -> Add2/2
  Y/1 -> Product6/2

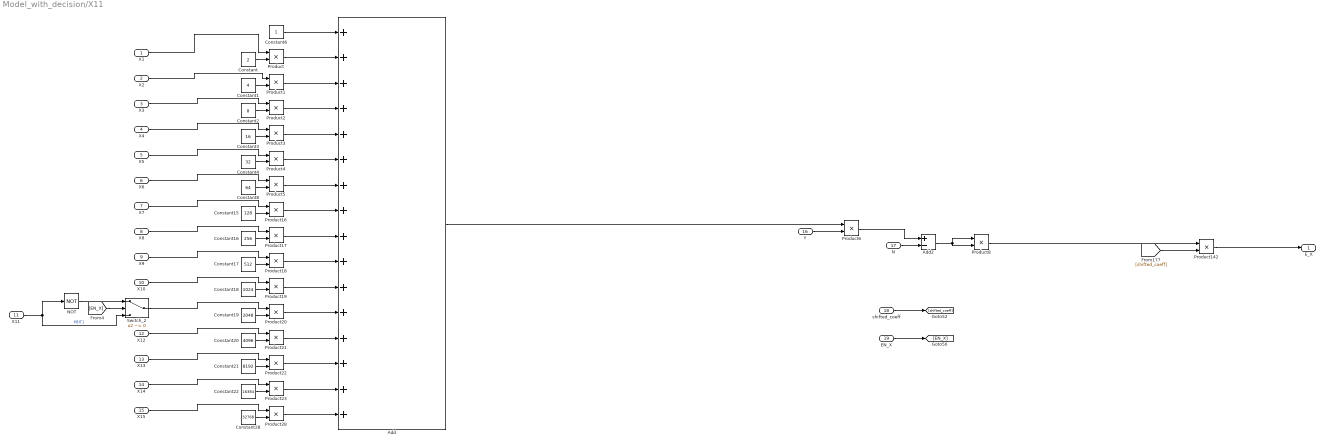
== system Model_with_decision/X11 ==
  X1 : Inport  OutDataTypeStr=fixdt(0,1,0)  LockScale=on
  X2 : Inport  Port=2  OutDataTypeStr=fixdt(0,1,0)  LockScale=on
  X3 : Inport  Port=3  OutDataTypeStr=fixdt(0,1,0)  LockScale=on
  X4 : Inport  Port=4  OutDataTypeStr=fixdt(0,1,0)  LockScale=on
  X5 : Inport  Port=5  OutDataTypeStr=fixdt(0,1,0)  LockScale=on
  X6 : Inport  Port=6  OutDataTypeStr=fixdt(0,1,0)  LockScale=on
  X7 : Inport  Port=7  OutDataTypeStr=fixdt(0,1,0)  LockScale=on
  X8 : Inport  Port=8  OutDataTypeStr=fixdt(0,1,0)  LockScale=on
  X9 : Inport  Port=9  OutDataTypeStr=fixdt(0,1,0)  LockScale=on
  X10 : Inport  Port=10  OutDataTypeStr=fixdt(0,1,0)  LockScale=on
  X11 : Inport  Port=11  OutDataTypeStr=fixdt(0,1,0)  LockScale=on
  X12 : Inport  Port=12  OutDataTypeStr=fixdt(0,1,0)  LockScale=on
  X13 : Inport  Port=13  OutDataTypeStr=fixdt(0,1,0)  LockScale=on
  X14 : Inport  Port=14  OutDataTypeStr=fixdt(0,1,0)  LockScale=on
  X15 : Inport  Port=15  OutDataTypeStr=fixdt(0,1,0)  LockScale=on
  Y : Inport  Port=16  LockScale=on
  N : Inport  Port=17  LockScale=on
  shifted_coeff : Inport  Port=18  LockScale=on
  EN_X : Inport  Port=19  OutDataTypeStr=fixdt(0,1,0)  LockScale=on
  Add : Sum  Inputs=++++++++++++++++
  Add2 : Sum  Inputs=+-
  Constant : Constant  Value=2
  Constant1 : Constant  Value=4
  Constant15 : Constant  Value=128
  Constant16 : Constant  Value=256
  Constant17 : Constant  Value=512
  Constant18 : Constant  Value=1024
  Constant19 : Constant  Value=2048
  Constant2 : Constant  Value=8
  Constant20 : Constant  Value=4096
  Constant21 : Constant  Value=8192
  Constant22 : Constant  Value=16384
  Constant28 : Constant  Value=32768
  Constant3 : Constant  Value=16
  Constant4 : Constant  Value=32
  Constant6 : Constant
  Constant8 : Constant  Value=64
  NOT : Logic  Operator=NOT  IconShape=distinctive  AllPortsSameDT=off  OutDataTypeStr=boolean
  Product{,1..6,8,16..23,28,142} (18 alike) : Product
  Switch_2 : Switch  Criteria=u2 ~= 0  OutDataTypeStr=fixdt(0,1,0)  SaturateOnIntegerOverflow=off  InputSameDT=off
  E_X : Outport  LockScale=on
  wires:
  Y/1 -> Product6/2
  N/1 -> Add2/2
  Product8/1 -> Product142/1
  Product6/1 -> Add2/1
  [shifted_coeff] -> Product142/2
  Product142/1 -> E_X/1
  shifted_coeff/1 -> [shifted_coeff]
  EN_X/1 -> [EN_X]
  X13/1 -> Product22/1
  NOT/1 -> Switch_2/1
  X11/1 -> NOT/1, Switch_2/3  "PBIT1"
  [EN_X] -> Switch_2/2
  Constant22/1 -> Product23/2
  Constant21/1 -> Product22/2
  Product23/1 -> Add/15
  Product22/1 -> Add/14
  Product28/1 -> Add/16
  Constant28/1 -> Product28/2
  X15/1 -> Product28/1
  X14/1 -> Product23/1
  Product17/1 -> Add/9
  X12/1 -> Product21/1
  Product21/1 -> Add/13
  Constant17/1 -> Product18/2
  X9/1 -> Product18/1
  Product16/1 -> Add/8
  Constant19/1 -> Product20/2
  X7/1 -> Product16/1
  X10/1 -> Product19/1
  X8/1 -> Product17/1
  Product20/1 -> Add/12
  Switch_2/1 -> Product20/1
  Constant16/1 -> Product17/2
  Constant15/1 -> Product16/2
  Product18/1 -> Add/10
  Constant18/1 -> Product19/2
  Constant20/1 -> Product21/2
  Product19/1 -> Add/11
  Constant3/1 -> Product3/2
  X5/1 -> Product4/1
  Product5/1 -> Add/7
  X4/1 -> Product3/1
  Product3/1 -> Add/5
  X6/1 -> Product5/1
  Constant8/1 -> Product5/2
  Constant4/1 -> Product4/2
  Product4/1 -> Add/6
  Add2/1 -> Product8/1, Product8/2
  Add/1 -> Product6/1
  Product2/1 -> Add/4
  Product1/1 -> Add/3
  Product/1 -> Add/2
  Constant6/1 -> Add/1
  X3/1 -> Product2/1
  Constant2/1 -> Product2/2
  X2/1 -> Product1/1
  Constant1/1 -> Product1/2
  X1/1 -> Product/1
  Constant/1 -> Product/2

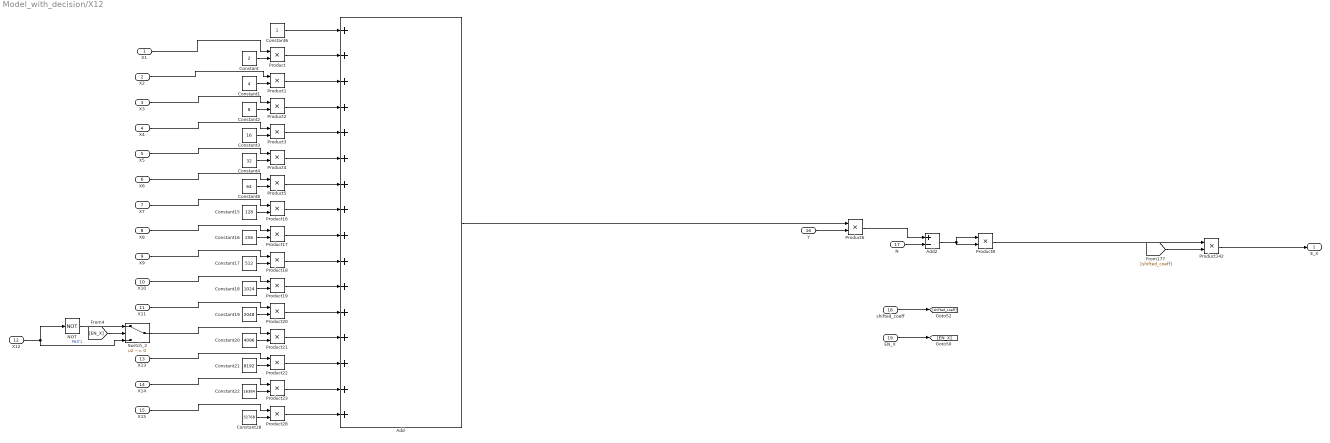
== system Model_with_decision/X12 ==
  X1 : Inport  OutDataTypeStr=fixdt(0,1,0)  LockScale=on
  X2 : Inport  Port=2  OutDataTypeStr=fixdt(0,1,0)  LockScale=on
  X3 : Inport  Port=3  OutDataTypeStr=fixdt(0,1,0)  LockScale=on
  X4 : Inport  Port=4  OutDataTypeStr=fixdt(0,1,0)  LockScale=on
  X5 : Inport  Port=5  OutDataTypeStr=fixdt(0,1,0)  LockScale=on
  X6 : Inport  Port=6  OutDataTypeStr=fixdt(0,1,0)  LockScale=on
  X7 : Inport  Port=7  OutDataTypeStr=fixdt(0,1,0)  LockScale=on
  X8 : Inport  Port=8  OutDataTypeStr=fixdt(0,1,0)  LockScale=on
  X9 : Inport  Port=9  OutDataTypeStr=fixdt(0,1,0)  LockScale=on
  X10 : Inport  Port=10  OutDataTypeStr=fixdt(0,1,0)  LockScale=on
  X11 : Inport  Port=11  OutDataTypeStr=fixdt(0,1,0)  LockScale=on
  X12 : Inport  Port=12  OutDataTypeStr=fixdt(0,1,0)  LockScale=on
  X13 : Inport  Port=13  OutDataTypeStr=fixdt(0,1,0)  LockScale=on
  X14 : Inport  Port=14  OutDataTypeStr=fixdt(0,1,0)  LockScale=on
  X15 : Inport  Port=15  OutDataTypeStr=fixdt(0,1,0)  LockScale=on
  Y : Inport  Port=16  LockScale=on
  N : Inport  Port=17  LockScale=on
  shifted_coeff : Inport  Port=18  LockScale=on
  EN_X : Inport  Port=19  OutDataTypeStr=fixdt(0,1,0)  LockScale=on
  Add : Sum  Inputs=++++++++++++++++
  Add2 : Sum  Inputs=+-
  Constant : Constant  Value=2
  Constant1 : Constant  Value=4
  Constant15 : Constant  Value=128
  Constant16 : Constant  Value=256
  Constant17 : Constant  Value=512
  Constant18 : Constant  Value=1024
  Constant19 : Constant  Value=2048
  Constant2 : Constant  Value=8
  Constant20 : Constant  Value=4096
  Constant21 : Constant  Value=8192
  Constant22 : Constant  Value=16384
  Constant28 : Constant  Value=32768
  Constant3 : Constant  Value=16
  Constant4 : Constant  Value=32
  Constant6 : Constant
  Constant8 : Constant  Value=64
  NOT : Logic  Operator=NOT  IconShape=distinctive  AllPortsSameDT=off  OutDataTypeStr=boolean
  Product{,1..6,8,16..23,28,142} (18 alike) : Product
  Switch_2 : Switch  Criteria=u2 ~= 0  OutDataTypeStr=fixdt(0,1,0)  SaturateOnIntegerOverflow=off  InputSameDT=off
  E_X : Outport  LockScale=on
  wires:
  Constant/1 -> Product/2
  X1/1 -> Product/1
  Constant1/1 -> Product1/2
  X2/1 -> Product1/1
  Constant2/1 -> Product2/2
  X3/1 -> Product2/1
  Constant6/1 -> Add/1
  Product/1 -> Add/2
  Product1/1 -> Add/3
  Product2/1 -> Add/4
  Add/1 -> Product6/1
  Add2/1 -> Product8/2, Product8/1
  Product4/1 -> Add/6
  Constant4/1 -> Product4/2
  Constant8/1 -> Product5/2
  X6/1 -> Product5/1
  Product3/1 -> Add/5
  X4/1 -> Product3/1
  Product5/1 -> Add/7
  X5/1 -> Product4/1
  Constant3/1 -> Product3/2
  Product19/1 -> Add/11
  Constant20/1 -> Product21/2
  Constant18/1 -> Product19/2
  Product18/1 -> Add/10
  Constant15/1 -> Product16/2
  Constant16/1 -> Product17/2
  X11/1 -> Product20/1
  Product20/1 -> Add/12
  X8/1 -> Product17/1
  X10/1 -> Product19/1
  X7/1 -> Product16/1
  Constant19/1 -> Product20/2
  Product16/1 -> Add/8
  X9/1 -> Product18/1
  Constant17/1 -> Product18/2
  Product21/1 -> Add/13
  Switch_2/1 -> Product21/1
  Product17/1 -> Add/9
  X14/1 -> Product23/1
  X15/1 -> Product28/1
  Constant28/1 -> Product28/2
  Product28/1 -> Add/16
  Product22/1 -> Add/14
  Product23/1 -> Add/15
  Constant21/1 -> Product22/2
  Constant22/1 -> Product23/2
  [EN_X] -> Switch_2/2
  X12/1 -> Switch_2/3, NOT/1  "PBIT1"
  NOT/1 -> Switch_2/1
  X13/1 -> Product22/1
  EN_X/1 -> [EN_X]
  shifted_coeff/1 -> [shifted_coeff]
  Product142/1 -> E_X/1
  [shifted_coeff] -> Product142/2
  Product6/1 -> Add2/1
  Product8/1 -> Product142/1
  N/1 -> Add2/2
  Y/1 -> Product6/2

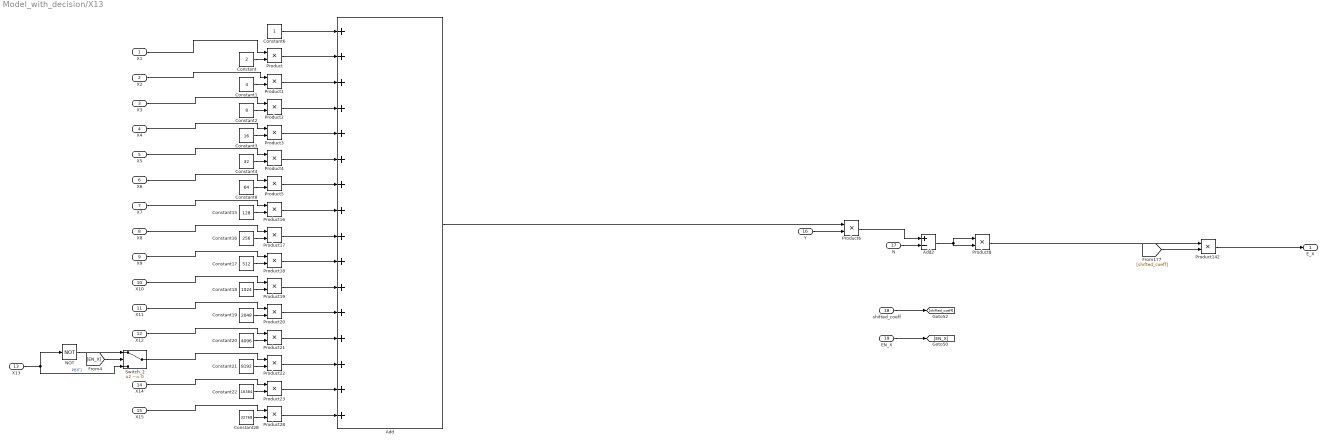
== system Model_with_decision/X13 ==
  X1 : Inport  OutDataTypeStr=fixdt(0,1,0)  LockScale=on
  X2 : Inport  Port=2  OutDataTypeStr=fixdt(0,1,0)  LockScale=on
  X3 : Inport  Port=3  OutDataTypeStr=fixdt(0,1,0)  LockScale=on
  X4 : Inport  Port=4  OutDataTypeStr=fixdt(0,1,0)  LockScale=on
  X5 : Inport  Port=5  OutDataTypeStr=fixdt(0,1,0)  LockScale=on
  X6 : Inport  Port=6  OutDataTypeStr=fixdt(0,1,0)  LockScale=on
  X7 : Inport  Port=7  OutDataTypeStr=fixdt(0,1,0)  LockScale=on
  X8 : Inport  Port=8  OutDataTypeStr=fixdt(0,1,0)  LockScale=on
  X9 : Inport  Port=9  OutDataTypeStr=fixdt(0,1,0)  LockScale=on
  X10 : Inport  Port=10  OutDataTypeStr=fixdt(0,1,0)  LockScale=on
  X11 : Inport  Port=11  OutDataTypeStr=fixdt(0,1,0)  LockScale=on
  X12 : Inport  Port=12  OutDataTypeStr=fixdt(0,1,0)  LockScale=on
  X13 : Inport  Port=13  OutDataTypeStr=fixdt(0,1,0)  LockScale=on
  X14 : Inport  Port=14  OutDataTypeStr=fixdt(0,1,0)  LockScale=on
  X15 : Inport  Port=15  OutDataTypeStr=fixdt(0,1,0)  LockScale=on
  Y : Inport  Port=16  LockScale=on
  N : Inport  Port=17  LockScale=on
  shifted_coeff : Inport  Port=18  LockScale=on
  EN_X : Inport  Port=19  OutDataTypeStr=fixdt(0,1,0)  LockScale=on
  Add : Sum  Inputs=++++++++++++++++
  Add2 : Sum  Inputs=+-
  Constant : Constant  Value=2
  Constant1 : Constant  Value=4
  Constant15 : Constant  Value=128
  Constant16 : Constant  Value=256
  Constant17 : Constant  Value=512
  Constant18 : Constant  Value=1024
  Constant19 : Constant  Value=2048
  Constant2 : Constant  Value=8
  Constant20 : Constant  Value=4096
  Constant21 : Constant  Value=8192
  Constant22 : Constant  Value=16384
  Constant28 : Constant  Value=32768
  Constant3 : Constant  Value=16
  Constant4 : Constant  Value=32
  Constant6 : Constant
  Constant8 : Constant  Value=64
  NOT : Logic  Operator=NOT  IconShape=distinctive  AllPortsSameDT=off  OutDataTypeStr=boolean
  Product{,1..6,8,16..23,28,142} (18 alike) : Product
  Switch_2 : Switch  Criteria=u2 ~= 0  OutDataTypeStr=fixdt(0,1,0)  SaturateOnIntegerOverflow=off  InputSameDT=off
  E_X : Outport  LockScale=on
  wires:
  Constant/1 -> Product/2
  X1/1 -> Product/1
  Constant1/1 -> Product1/2
  X2/1 -> Product1/1
  Constant2/1 -> Product2/2
  X3/1 -> Product2/1
  Constant6/1 -> Add/1
  Product/1 -> Add/2
  Product1/1 -> Add/3
  Product2/1 -> Add/4
  Add/1 -> Product6/1
  Add2/1 -> Product8/2, Product8/1
  Product4/1 -> Add/6
  Constant4/1 -> Product4/2
  Constant8/1 -> Product5/2
  X6/1 -> Product5/1
  Product3/1 -> Add/5
  X4/1 -> Product3/1
  Product5/1 -> Add/7
  X5/1 -> Product4/1
  Constant3/1 -> Product3/2
  Product19/1 -> Add/11
  Constant20/1 -> Product21/2
  Constant18/1 -> Product19/2
  Product18/1 -> Add/10
  Constant15/1 -> Product16/2
  Constant16/1 -> Product17/2
  X11/1 -> Product20/1
  Product20/1 -> Add/12
  X8/1 -> Product17/1
  X10/1 -> Product19/1
  X7/1 -> Product16/1
  Constant19/1 -> Product20/2
  Product16/1 -> Add/8
  X9/1 -> Product18/1
  Constant17/1 -> Product18/2
  Product21/1 -> Add/13
  X12/1 -> Product21/1
  Product17/1 -> Add/9
  X14/1 -> Product23/1
  X15/1 -> Product28/1
  Constant28/1 -> Product28/2
  Product28/1 -> Add/16
  Product22/1 -> Add/14
  Product23/1 -> Add/15
  Constant21/1 -> Product22/2
  Constant22/1 -> Product23/2
  [EN_X] -> Switch_2/2
  X13/1 -> NOT/1, Switch_2/3  "PBIT1"
  NOT/1 -> Switch_2/1
  Switch_2/1 -> Product22/1
  EN_X/1 -> [EN_X]
  shifted_coeff/1 -> [shifted_coeff]
  Product142/1 -> E_X/1
  [shifted_coeff] -> Product142/2
  Product6/1 -> Add2/1
  Product8/1 -> Product142/1
  N/1 -> Add2/2
  Y/1 -> Product6/2
